simulink model "atrias_original"  (R2017a)
settings: Solver=ode45  StartTime=0.0  StopTime=sim_t  RelTol=1e-6  EnableMultiTasking=on
values from neighbouring files (symbols this model uses):
  N = grid_slice*1000    [createGrid.m]
  nm = fn_set_vnmc_params(sm, sample_time)    [kernel_scores_NM_mismatch.m]    (also in main_ATRIAS_cluster.m)
  nmc_BLCtrlPar = nmc.BLCtrlPar    [kernel_scores_NM_mismatch.m]    (also in main_ATRIAS_cluster.m)
  nmc_FPCtrlPar = nmc.FPCtrlPar    [kernel_scores_NM_mismatch.m]    (also in main_ATRIAS_cluster.m)
  nmc_LLCtrlPar = nmc.LLCtrlPar    [kernel_scores_NM_mismatch.m]    (also in main_ATRIAS_cluster.m)
  nmc_StCtrlPar = nmc.StCtrlPar    [kernel_scores_NM_mismatch.m]    (also in main_ATRIAS_cluster.m)
  nmc_SwCtrlPar = nmc.SwCtrlPar    [kernel_scores_NM_mismatch.m]    (also in main_ATRIAS_cluster.m)
  nmc_TrCtrlPar = nmc.TrCtrlPar    [kernel_scores_NM_mismatch.m]    (also in main_ATRIAS_cluster.m)
  nStep_switchCtrl = 10    [main_ATRIAS_cluster.m]
  nStep_thr = 1000    [createSimInitial.m]    (also in main_ATRIAS_cluster.m)
  rc_CtrlPar = [rc.k_placement, rc.T_step, rc.Cd, rc.kpt, rc.kdt, rc.desired_theta, rc.desired_z, rc.kpz, rc.kdz]    [kernel_scores_NM_mismatch.m]    (also in main_ATRIAS_cluster.m)
  sm = fn_set_MechParams(sm)    [kernel_scores_NM_mismatch.m]    (also in main_ATRIAS_cluster.m = fn_set_MechParams(sm,perturb))
  test_VNMC = 1    [createSimInitial.m]    (also in main_ATRIAS_cluster.m = 0)
undefined symbols (not defined in the file or in its folder): delta_phi_max, delta_phi_max_buffer, delta_phi_min, DiscIntNeverNeededParam, Discrete, idc, initial_dx_estimate, initial_dy_estimate, initial_dz_estimate, initial_z_estimate, kd_shin_max, kd_shin_min, kd_splay_max, kd_splay_min, kd_thigh_max, kd_thigh_min, kp_shin_max, kp_shin_min, kp_splay_max, kp_splay_min, kp_thigh_max, kp_thigh_min, mc, min_splay_angle, min_splay_buffer, phi_shin_max, phi_shin_max_buffer, phi_shin_min, phi_shin_min_buffer, phi_thigh_max, phi_thigh_max_buffer, phi_thigh_min, phi_thigh_min_buffer, rad, rc, s, sample_time, sgn, sim_d, t_friction, Time, X, Y, Z
libraries: sm_lib x202, nesl_utility x122, simulink x77, simulink_extras x24, fl_lib x16, mblibv1 x4, ctrlSharedLib x4, commnoisgen2 x1, dspswit3 x1
(part 8 of 17)

== system atrias_original/ATRIAS_sim/Mechanical System Layer/R Hip Shaft/Frame Data ==
  Kinematic Data : ToWorkspace  VariableName=r_hip_out  SampleTime=sm.output_sample_time
      settings: Save2DSignal=2-D array (concatenate along first dimension)
  Mux : Mux
  PS-Simulink Converter{,1..3} (4 alike) : nesl_utility/PS-Simulink Converter  PhysicalDomain=network_engine_domain  SubClassName=ps_output  LeftPortType=input  RightPortType=output  PseudoPeriodic=off  Frequencies=[]  Unit=1  AffineConversion=off
  Transform Sensor : sm_lib/Frames and Transforms/Transform Sensor  MeasurementFrame=World  SenseAngle=off  SenseAxis=off  SenseAngle1=off  SenseAngle2=off  SenseAngle3=off  SenseQ=on  SenseR=off  SenseOmegaX=off  SenseOmegaY=off  SenseOmegaZ=off  SenseOmega1=off  SenseOmega2=off  SenseOmega3=off  SenseQDot=off  SenseRDot=off  SenseAlphaX=off  SenseAlphaY=off  SenseAlphaZ=off  SenseAlpha1=off  SenseAlpha2=off  SenseAlpha3=off  SenseQDDot=off  SenseRDDot=off  SenseX=on  SenseY=on  SenseZ=on  SenseRad=off  SenseAzim=off  SenseDist=off  SenseInc=off  SenseXDot=off  SenseYDot=off  SenseZDot=off  SenseRadDot=off  SenseAzimDot=off  SenseDistDot=off  SenseIncDot=off  SenseXDDot=off  SenseYDDot=off  SenseZDDot=off  SenseRadDDot=off  SenseAzimDDot=off  SenseDistDDot=off  SenseIncDDot=off
  World Frame : sm_lib/Frames and Transforms/World Frame
  Frame : PMIOPort  Port=1  Side=Left
  wires:
  Mux/1 -> Kinematic Data/1
  PS-Simulink Converter/1 -> Mux/1
  PS-Simulink Converter1/1 -> Mux/2
  PS-Simulink Converter2/1 -> Mux/3
  PS-Simulink Converter3/1 -> Mux/4
  connections:
  PS-Simulink Converter3/LConn1 -- Transform Sensor/RConn5
  PS-Simulink Converter2/LConn1 -- Transform Sensor/RConn4
  PS-Simulink Converter1/LConn1 -- Transform Sensor/RConn3
  PS-Simulink Converter/LConn1 -- Transform Sensor/RConn2
  Transform Sensor/RConn1 -- Frame/RConn1
  Transform Sensor/LConn1 -- World Frame/RConn1

== system atrias_original/ATRIAS_sim/Mechanical System Layer/R Leg/Angle Range Map ==
  "[-pi, pi]" : Inport
  Constant : Constant  Value=2*pi
  Sum3 : Sum  Inputs=|++
  Switch : Switch  ZeroCross=off
  "[0,2*pi]" : Outport
  wires:
  "[-pi, pi]"/1 -> Sum3/1, Switch/1, Switch/2
  Sum3/1 -> Switch/3
  Constant/1 -> Sum3/2
  Switch/1 -> "[0,2*pi]"/1

== system atrias_original/ATRIAS_sim/Mechanical System Layer/R Leg/Angle Range Map1 ==
  "[-pi, pi]" : Inport
  Constant : Constant  Value=2*pi
  Sum3 : Sum  Inputs=|++
  Switch : Switch  ZeroCross=off
  "[0,2*pi]" : Outport
  wires:
  Switch/1 -> "[0,2*pi]"/1
  Constant/1 -> Sum3/2
  Sum3/1 -> Switch/3
  "[-pi, pi]"/1 -> Switch/2, Switch/1, Sum3/1

== system atrias_original/ATRIAS_sim/Mechanical System Layer/R Leg/Four Bar Link ==
  CS1 to CS2 : sm_lib/Frames and Transforms/Rigid Transform  TranslationMethod=Cartesian  TranslationStandardOffset=0  TranslationLengthUnit=m  TranslationStandardAxis=+Z  TranslationCartesianOffset=[0 -sm.l_seg 0]  TranslationROffset=0  TranslationROffsetUnits=m  TranslationZOffset=0  TranslationZOffsetUnits=m  TranslationThetaOffset=0  TranslationThetaOffsetUnits=deg  RotationMethod=None  RotationAngleUnits=deg  RotationStandardAxis=+Z  RotationAngle=0  RotationArbitraryAxis=[0 0 1]  FollAlignAxisA=+X  BaseAlignAxisA=+Y  FollAlignAxisB=+Y  BaseAlignAxisB=+Z  RotationSequenceAxes=FollowerAxes  RotationSequence=XYX  RotationSequenceAngles=[0 0 0]  RotationSequenceAnglesUnits=deg  RotationMatrix=[1 0 0; 0 1 0; 0 0 1]
  Frame Data : Subsystem
  Solid : sm_lib/Body Elements/Solid  InertiaType=Custom  Mass=sm.m_fblink  MassUnits=kg  CenterOfMass=sm.com_fblink  CenterOfMassUnits=m  MomentsOfInertia=sm.i_fblink_moments  MomentsOfInertiaUnits=kg*m^2  ProductsOfInertia=sm.i_fblink_products  ProductsOfInertiaUnits=kg*m^2  DensityBased=on  Density=1000  DensityUnits=kg/(m^3)  DoExposeReferenceFrame=on  SerializedFrames=<Frames/>  GraphicType=FromGeometry  MarkerShape=Sphere  MarkerSize=10  MarkerSizeUnits=m  GraphicVisPropType=AdvancedVisualProperties  GraphicDiffuseColor=sm.fblink_color_d  GraphicSpecularColor=[0.5 0.5 0.5 1.0]  GraphicAmbientColor=[sm.fblink_color_d*0.5 1.0]  GraphicEmissiveColor=[0.0 0.0 0.0 1.0]  GraphicShininess=128  GraphicOpacity=1.0  GeometryShape=FromFile  RectangleSize=[1 1]  RectangleSizeUnits=m  BrickDimensions="[0.1  1 0.1]"  BrickDimensionUnits=m  CylinderRadius=1  CylinderRadiusUnits=m  CylinderLength=1  CylinderLengthUnits=m  SphereRadius=1  SphereRadiusUnits=m  EllipsoidRadii=[1 1 1]  EllipsoidRadiiUnits=m  ExtrusionCrossSection=[1 1; -1 1; -1 -1; 1 -1]  ExtrusionCrossSectionUnits=m  ExtrusionLength=1  ExtrusionLengthUnits=m  PolygonNumSides=3  PolygonOuterRadius=1  PolygonOuterRadiusUnits=m  ExtGeomFileType=STL  ExtGeomFileName=../models/four_bar_link.stl  ExtGeomFileUnits=m  RevolutionCrossSection=[1 1; 1 -1; 2 -1; 2 1]  RevolutionCrossSectionUnits=m  RevolutionExtent=Full  RevolutionAngle=180  RevolutionAngleUnits=deg
  CS1 : PMIOPort  Port=1  Side=Left
  CS2 : PMIOPort  Port=2  Side=Right
  connections:
  CS2/RConn1 -- CS1 to CS2/RConn1
  Solid/RConn1 -- CS1/RConn1 -- Frame Data/LConn1 -- CS1 to CS2/LConn1

== system atrias_original/ATRIAS_sim/Mechanical System Layer/R Leg/Lower Leg ==
  CS1 to CS2 : sm_lib/Frames and Transforms/Rigid Transform  TranslationMethod=Cartesian  TranslationStandardOffset=0  TranslationLengthUnit=m  TranslationStandardAxis=+Z  TranslationCartesianOffset=[0 -sm.lowerleg_12 0]  TranslationROffset=0  TranslationROffsetUnits=m  TranslationZOffset=0  TranslationZOffsetUnits=m  TranslationThetaOffset=0  TranslationThetaOffsetUnits=deg  RotationMethod=None  RotationAngleUnits=deg  RotationStandardAxis=+Z  RotationAngle=0  RotationArbitraryAxis=[0 0 1]  FollAlignAxisA=+X  BaseAlignAxisA=+Y  FollAlignAxisB=+Y  BaseAlignAxisB=+Z  RotationSequenceAxes=FollowerAxes  RotationSequence=XYX  RotationSequenceAngles=[0 0 0]  RotationSequenceAnglesUnits=deg  RotationMatrix=[1 0 0; 0 1 0; 0 0 1]
  CS1 to CS3 : sm_lib/Frames and Transforms/Rigid Transform  TranslationMethod=Cartesian  TranslationStandardOffset=0  TranslationLengthUnit=m  TranslationStandardAxis=+Z  TranslationCartesianOffset=[0 -sm.l_seg 0]  TranslationROffset=0  TranslationROffsetUnits=m  TranslationZOffset=0  TranslationZOffsetUnits=m  TranslationThetaOffset=0  TranslationThetaOffsetUnits=deg  RotationMethod=None  RotationAngleUnits=deg  RotationStandardAxis=+Z  RotationAngle=0  RotationArbitraryAxis=[0 0 1]  FollAlignAxisA=+X  BaseAlignAxisA=+Y  FollAlignAxisB=+Y  BaseAlignAxisB=+Z  RotationSequenceAxes=FollowerAxes  RotationSequence=XYX  RotationSequenceAngles=[0 0 0]  RotationSequenceAnglesUnits=deg  RotationMatrix=[1 0 0; 0 1 0; 0 0 1]
  Frame Data : Subsystem
  Solid : sm_lib/Body Elements/Solid  InertiaType=Custom  Mass=sm.m_lowerleg  MassUnits=kg  CenterOfMass=sm.com_lowerleg  CenterOfMassUnits=m  MomentsOfInertia=sm.i_lowerleg_moments  MomentsOfInertiaUnits=kg*m^2  ProductsOfInertia=sm.i_lowerleg_products  ProductsOfInertiaUnits=kg*m^2  DensityBased=on  Density=1000  DensityUnits=kg/(m^3)  DoExposeReferenceFrame=on  SerializedFrames=<Frames/>  GraphicType=FromGeometry  MarkerShape=Sphere  MarkerSize=10  MarkerSizeUnits=m  GraphicVisPropType=AdvancedVisualProperties  GraphicDiffuseColor=sm.lowerleg_color_d  GraphicSpecularColor=[0.5 0.5 0.5 1.0]  GraphicAmbientColor=[sm.lowerleg_color_d*0.5 1.0]  GraphicEmissiveColor=[0.0 0.0 0.0 1.0]  GraphicShininess=128  GraphicOpacity=1.0  GeometryShape=FromFile  RectangleSize=[1 1]  RectangleSizeUnits=m  BrickDimensions=[0.1 1 0.1]  BrickDimensionUnits=m  CylinderRadius=1  CylinderRadiusUnits=m  CylinderLength=1  CylinderLengthUnits=m  SphereRadius=1  SphereRadiusUnits=m  EllipsoidRadii=[1 1 1]  EllipsoidRadiiUnits=m  ExtrusionCrossSection=[1 1; -1 1; -1 -1; 1 -1]  ExtrusionCrossSectionUnits=m  ExtrusionLength=1  ExtrusionLengthUnits=m  PolygonNumSides=3  PolygonOuterRadius=1  PolygonOuterRadiusUnits=m  ExtGeomFileType=STL  ExtGeomFileName=../models/lower_leg.stl  ExtGeomFileUnits=m  RevolutionCrossSection=[1 1; 1 -1; 2 -1; 2 1]  RevolutionCrossSectionUnits=m  RevolutionExtent=Full  RevolutionAngle=180  RevolutionAngleUnits=deg
  CS1 : PMIOPort  Port=1  Side=Left
  CS2 : PMIOPort  Port=2  Side=Right
  CS3 : PMIOPort  Port=3  Side=Right
  connections:
  CS3/RConn1 -- CS1 to CS3/RConn1
  CS1 to CS3/LConn1 -- CS1 to CS2/LConn1 -- Solid/RConn1 -- Frame Data/LConn1 -- CS1/RConn1
  CS2/RConn1 -- CS1 to CS2/RConn1

== system atrias_original/ATRIAS_sim/Mechanical System Layer/R Leg/Mechanical Limits ==
  note: Thigh-Shin Flexion Collision
  note: Thigh-Shin Collision
  note: Mechanical Limits Model
  dphi_shin : Inport
  phi_shin : Inport  Port=2
  dphi_thigh : Inport  Port=3
  phi_thigh : Inport  Port=4
  Compare To Constant5 : simulink/Logic and Bit Operations/Compare To Constant  relop=<=  const=sm.phi_max_collision  OutDataTypeStr=boolean  ZeroCross=off
  Compare To Zero{,1..5} (6 alike) : simulink/Logic and Bit Operations/Compare To Zero  relop=<=  OutDataTypeStr=boolean  ZeroCross=off
  Constant : Constant  Value=sm.delta_phi_min
  Constant1 : Constant  Value=sm.phi_shin_max
  Constant2 : Constant  Value=sm.phi_thigh_min
  Constant3 : Constant  Value=sm.delta_phi_max
  Constant4 : Constant  Value=sm.phi_shin_min
  Constant5 : Constant  Value=sm.phi_thigh_max
  Enabled Subsystem : Subsystem  TreatAsAtomicUnit=on
  Gain : Gain  Gain=-1
  Gain1 : Gain  Gain=-1
  Gain2 : Gain  Gain=-1
  Logical Operator : Logic  Operator=OR  Inputs=1  AllPortsSameDT=off  OutDataTypeStr=boolean
  Mux : Mux  Inputs=6
  Shin Max Collision Model : Subsystem
  Shin Min Collision Model : Subsystem
  Stop Simulation6 : Stop
  Sum{1..3,5,7} (5 alike) : Sum  Inputs=-+|
  Sum10 : Sum  Inputs=+-|
  Sum11 : Sum  Inputs=-|+
  Sum4 : Sum  Inputs=+-|
  Sum6 : Sum  Inputs=+|-
  Sum8 : Sum  Inputs=+-|
  Sum9 : Sum  Inputs=-|+
  Thigh Max Collision Model : Subsystem
  Thigh Min Collision Model : Subsystem
  Thigh-Shin Collision Model : Subsystem
  Thigh-Shin Collision Model1 : Subsystem
  tau_shin_col : Outport
  tau_thigh_shin_col : Outport  Port=2
  tau_thigh_col : Outport  Port=3
  wires:
  Compare To Constant5/1 -> Logical Operator/1, Enabled Subsystem/1(Col_Flags)
  Sum4/1 -> Shin Max Collision Model/1(phi [rad]), Compare To Zero1/1, [col_r_shin_max]
  Sum10/1 -> [col_r_thigh_max], Compare To Zero5/1, Thigh Max Collision Model/1(phi [rad])
  Logical Operator/1 -> Enabled Subsystem/Enable, Stop Simulation6/1
  Mux/1 -> Compare To Constant5/1
  [col_r_leg_flexion] -> Mux/6
  [col_r_leg_extension] -> Mux/5
  [col_r_shin_min] -> Mux/4
  [col_r_shin_max] -> Mux/3
  [col_r_thigh_min] -> Mux/2
  [col_r_thigh_max] -> Mux/1
  Thigh Max Collision Model/1(tau_interaction[Nm]) -> Sum11/1
  Gain1/1 -> Thigh Max Collision Model/2(vphi [rad/s])
  Thigh Min Collision Model/1(tau_interaction[Nm]) -> Sum11/2
  Sum11/1 -> tau_thigh_col/1
  Compare To Zero5/1 -> Thigh Max Collision Model/Enable
  Constant5/1 -> Sum10/1
  Sum6/1 -> tau_thigh_shin_col/1
  Shin Min Collision Model/1(tau_interaction[Nm]) -> Sum9/2
  Shin Max Collision Model/1(tau_interaction[Nm]) -> Sum9/1
  Sum9/1 -> tau_shin_col/1
  dphi_shin/1 -> Shin Min Collision Model/2(vphi [rad/s]), Gain/1, Sum2/2
  Sum7/1 -> Shin Min Collision Model/1(phi [rad]), Compare To Zero4/1, [col_r_shin_min]
  Constant4/1 -> Sum7/1
  Compare To Zero4/1 -> Shin Min Collision Model/Enable
  Gain2/1 -> Thigh-Shin Collision Model1/2(vphi [rad/s])
  Thigh-Shin Collision Model1/1(tau_interaction[Nm]) -> Sum6/2
  Thigh-Shin Collision Model/1(tau_interaction[Nm]) -> Sum6/1
  Sum8/1 -> Thigh-Shin Collision Model1/1(delta_phi [rad]), Compare To Zero3/1, [col_r_leg_flexion]
  Constant3/1 -> Sum8/1
  Compare To Zero3/1 -> Thigh-Shin Collision Model1/Enable
  Compare To Zero2/1 -> Thigh Min Collision Model/Enable
  Gain/1 -> Shin Max Collision Model/2(vphi [rad/s])
  Sum5/1 -> Thigh Min Collision Model/1(phi [rad]), Compare To Zero2/1, [col_r_thigh_min]
  Constant2/1 -> Sum5/1
  dphi_thigh/1 -> Sum2/1, Gain1/1, Thigh Min Collision Model/2(vphi [rad/s])
  phi_thigh/1 -> Sum1/1, Sum5/2, Sum10/2
  Constant1/1 -> Sum4/1
  Compare To Zero1/1 -> Shin Max Collision Model/Enable
  Sum3/1 -> Thigh-Shin Collision Model/1(delta_phi [rad]), Compare To Zero/1, [col_r_leg_extension]
  Constant/1 -> Sum3/1
  Sum2/1 -> Thigh-Shin Collision Model/2(vphi [rad/s]), Gain2/1
  phi_shin/1 -> Sum4/2, Sum7/2, Sum1/2
  Sum1/1 -> Sum3/2, Sum8/2
  Compare To Zero/1 -> Thigh-Shin Collision Model/Enable

== system atrias_original/ATRIAS_sim/Mechanical System Layer/R Leg/Shin ==
  CS1 to CS2 : sm_lib/Frames and Transforms/Rigid Transform  TranslationMethod=Cartesian  TranslationStandardOffset=0  TranslationLengthUnit=m  TranslationStandardAxis=+Z  TranslationCartesianOffset=[0 -sm.shin_12 0]  TranslationROffset=0  TranslationROffsetUnits=m  TranslationZOffset=0  TranslationZOffsetUnits=m  TranslationThetaOffset=0  TranslationThetaOffsetUnits=deg  RotationMethod=None  RotationAngleUnits=deg  RotationStandardAxis=+Z  RotationAngle=0  RotationArbitraryAxis=[0 0 1]  FollAlignAxisA=+X  BaseAlignAxisA=+Y  FollAlignAxisB=+Y  BaseAlignAxisB=+Z  RotationSequenceAxes=FollowerAxes  RotationSequence=XYX  RotationSequenceAngles=[0 0 0]  RotationSequenceAnglesUnits=deg  RotationMatrix=[1 0 0; 0 1 0; 0 0 1]
  Frame Data : Subsystem
  Solid : sm_lib/Body Elements/Solid  InertiaType=Custom  Mass=sm.m_shin  MassUnits=kg  CenterOfMass=sm.com_shin  CenterOfMassUnits=m  MomentsOfInertia=sm.i_shin_moments  MomentsOfInertiaUnits=kg*m^2  ProductsOfInertia=sm.i_shin_products  ProductsOfInertiaUnits=kg*m^2  DensityBased=on  Density=1000  DensityUnits=kg/(m^3)  DoExposeReferenceFrame=on  SerializedFrames=<Frames/>  GraphicType=FromGeometry  MarkerShape=Sphere  MarkerSize=10  MarkerSizeUnits=m  GraphicVisPropType=AdvancedVisualProperties  GraphicDiffuseColor=sm.shin_color_d  GraphicSpecularColor=[0.5 0.5 0.5 1.0]  GraphicAmbientColor=[sm.shin_color_d*0.5 1.0]  GraphicEmissiveColor=[0.0 0.0 0.0 1.0]  GraphicShininess=128  GraphicOpacity=1.0  GeometryShape=FromFile  RectangleSize=[1 1]  RectangleSizeUnits=m  BrickDimensions=[1 1 1]  BrickDimensionUnits=m  CylinderRadius=1  CylinderRadiusUnits=m  CylinderLength=1  CylinderLengthUnits=m  SphereRadius=1  SphereRadiusUnits=m  EllipsoidRadii=[1 1 1]  EllipsoidRadiiUnits=m  ExtrusionCrossSection=[1 1; -1 1; -1 -1; 1 -1]  ExtrusionCrossSectionUnits=m  ExtrusionLength=1  ExtrusionLengthUnits=m  PolygonNumSides=3  PolygonOuterRadius=1  PolygonOuterRadiusUnits=m  ExtGeomFileType=STL  ExtGeomFileName=../models/shin.stl  ExtGeomFileUnits=m  RevolutionCrossSection=[1 1; 1 -1; 2 -1; 2 1]  RevolutionCrossSectionUnits=m  RevolutionExtent=Full  RevolutionAngle=180  RevolutionAngleUnits=deg
  CS1 : PMIOPort  Port=1  Side=Left
  CS2 : PMIOPort  Port=2  Side=Right
  connections:
  CS1 to CS2/LConn1 -- CS1/RConn1 -- Frame Data/LConn1 -- Solid/RConn1
  CS2/RConn1 -- CS1 to CS2/RConn1

== system atrias_original/ATRIAS_sim/Mechanical System Layer/R Leg/Shin SEA ==
  note: Shin SEA Mechanics
  Shin Gear Torque [Nm] : Inport
  Shin Joint [rad rad/s] : Inport  Port=2
  Continuous Angle : mblibv1/Utilities/Continuous Angle  rad=rad  rads=rad/s
      settings: SourceProductName=Simscape Multibody  SourceProductBaseCode=MS
  Demux : Demux  Outputs=2
  Gain : Gain  Gain=sm.k_leg_spring
  Gain1 : Gain  Gain=sm.b_leg_spring
  Initial Gear Angle : Constant  Value=sm.shin_initial_r
  Inverse Gear Ratio1 : Gain  Gain=1/sm.N
  Inverse Gear Ratio2 : Gain  Gain=sm.Kt_leg
  Inverse Gear Ratio3 : Gain  Gain=1/sm.Kt_leg
  Motor Direction : Gain  Gain=-1
  Motor Efficiency : Gain  Gain=sm.mu_motor
  Motor Controller : Subsystem  Commented=on
  Motor Electromagnetism : Subsystem  Commented=on
  Rotor Damping : Gain  Gain=sm.b_rotor
  Rotor and Gearing : Subsystem
  Sum : Sum  Inputs=++|
  Sum2 : Sum  Inputs=+|-
  Sum3 : Sum  Inputs=|+-
  Sum4 : Sum  Inputs=+|-
  Sum5 : Sum  Inputs=|++
  Torque Limiter (outside) 2 : Saturate  UpperLimit=sm.LEG_MTR_MAX_TORQUE  LowerLimit=-sm.LEG_MTR_MAX_TORQUE  ZeroCross=off
      settings: AttributesFormatString=Hi: %<UpperLimit>\nLo: %<LowerLimit>
  Rotor Joint Conn : PMIOPort  Port=1  Side=Left
  Shin Joint Torque [Nm] : Outport
  Shin Gear [rad] : Outport  Port=2
  wires:
  Sum2/1 -> Gain/1
  Gain/1 -> Sum5/1  "tau_load"
  Gain1/1 -> Sum5/2
  Sum4/1 -> Gain1/1
  Shin Joint [rad rad/s]/1 -> Demux/1
  Demux/1 -> Sum2/2
  Demux/2 -> Sum4/2
  Initial Gear Angle/1 -> Sum/1
  Sum/1 -> Sum2/1, Shin Gear [rad]/1
  Shin Gear Torque [Nm]/1 -> Motor Direction/1
  Sum3/1 -> Motor Efficiency/1
  Rotor Damping/1 -> Sum3/2
  Inverse Gear Ratio3/1 -> Inverse Gear Ratio2/1
  Inverse Gear Ratio2/1 -> Sum3/1
  Motor Controller/1(Voltage [V]) -> Motor Electromagnetism/1(Voltage [V])
  Motor Electromagnetism/1(Current [A]) -> Motor Controller/2(Measured Current [A])
  Inverse Gear Ratio1/1 -> Inverse Gear Ratio3/1
  Motor Efficiency/1 -> Rotor and Gearing/1(Rotor Torque [Nm])
  Rotor and Gearing/3(Rotor Velocity [rad/s]) -> Rotor Damping/1
  Torque Limiter (outside) 2/1 -> Inverse Gear Ratio1/1
  Sum5/1 -> Rotor and Gearing/2(Spring Torque [Nm]), Shin Joint Torque [Nm]/1
  Rotor and Gearing/1(Gearhead Position [rad]) -> Continuous Angle/1
  Rotor and Gearing/2(Gearhead Velocity [rad/s]) -> Sum4/1, Continuous Angle/2
  Continuous Angle/1 -> Sum/2
  Motor Direction/1 -> Torque Limiter (outside) 2/1
  connections:
  Rotor and Gearing/LConn1 -- Rotor Joint Conn/RConn1

== system atrias_original/ATRIAS_sim/Mechanical System Layer/R Leg/Thigh ==
  CS1 to CS2 : sm_lib/Frames and Transforms/Rigid Transform  TranslationMethod=Cartesian  TranslationStandardOffset=0  TranslationLengthUnit=m  TranslationStandardAxis=+Z  TranslationCartesianOffset=[0 -sm.l_seg 0]  TranslationROffset=0  TranslationROffsetUnits=m  TranslationZOffset=0  TranslationZOffsetUnits=m  TranslationThetaOffset=0  TranslationThetaOffsetUnits=deg  RotationMethod=None  RotationAngleUnits=deg  RotationStandardAxis=+Z  RotationAngle=0  RotationArbitraryAxis=[0 0 1]  FollAlignAxisA=+X  BaseAlignAxisA=+Y  FollAlignAxisB=+Y  BaseAlignAxisB=+Z  RotationSequenceAxes=FollowerAxes  RotationSequence=XYX  RotationSequenceAngles=[0 0 0]  RotationSequenceAnglesUnits=deg  RotationMatrix=[1 0 0; 0 1 0; 0 0 1]
  Frame Data : Subsystem
  Solid : sm_lib/Body Elements/Solid  InertiaType=Custom  Mass=sm.m_thigh  MassUnits=kg  CenterOfMass=sm.com_thigh  CenterOfMassUnits=m  MomentsOfInertia=sm.i_thigh_moments  MomentsOfInertiaUnits=kg*m^2  ProductsOfInertia=sm.i_thigh_products  ProductsOfInertiaUnits=kg*m^2  DensityBased=on  Density=1000  DensityUnits=kg/(m^3)  DoExposeReferenceFrame=on  SerializedFrames=<Frames/>  GraphicType=FromGeometry  MarkerShape=Sphere  MarkerSize=10  MarkerSizeUnits=m  GraphicVisPropType=AdvancedVisualProperties  GraphicDiffuseColor=sm.thigh_color_d  GraphicSpecularColor=[0.5 0.5 0.5 1.0]  GraphicAmbientColor=[sm.thigh_color_d*0.5 1.0]  GraphicEmissiveColor=[0.0 0.0 0.0 1.0]  GraphicShininess=128  GraphicOpacity=1.0  GeometryShape=FromFile  RectangleSize=[1 1]  RectangleSizeUnits=m  BrickDimensions=[1 1 1]  BrickDimensionUnits=m  CylinderRadius=1  CylinderRadiusUnits=m  CylinderLength=1  CylinderLengthUnits=m  SphereRadius=1  SphereRadiusUnits=m  EllipsoidRadii=[1 1 1]  EllipsoidRadiiUnits=m  ExtrusionCrossSection=[1 1; -1 1; -1 -1; 1 -1]  ExtrusionCrossSectionUnits=m  ExtrusionLength=1  ExtrusionLengthUnits=m  PolygonNumSides=3  PolygonOuterRadius=1  PolygonOuterRadiusUnits=m  ExtGeomFileType=STL  ExtGeomFileName=../models/thigh.stl  ExtGeomFileUnits=m  RevolutionCrossSection=[1 1; 1 -1; 2 -1; 2 1]  RevolutionCrossSectionUnits=m  RevolutionExtent=Full  RevolutionAngle=180  RevolutionAngleUnits=deg
  CS1 : PMIOPort  Port=1  Side=Left
  CS2 : PMIOPort  Port=2  Side=Right
  connections:
  CS2/RConn1 -- CS1 to CS2/RConn1
  CS1 to CS2/LConn1 -- Solid/RConn1 -- Frame Data/LConn1 -- CS1/RConn1

== system atrias_original/ATRIAS_sim/Mechanical System Layer/R Leg/Thigh SEA ==
  note: Thigh SEA Mechanics
  Thigh Gear Torque [Nm] : Inport
  Thigh Joint [rad rad/s] : Inport  Port=2
  Continuous Angle : mblibv1/Utilities/Continuous Angle  rad=rad  rads=rad/s
      settings: SourceProductName=Simscape Multibody  SourceProductBaseCode=MS
  Demux : Demux  Outputs=2
  Gain : Gain  Gain=sm.k_leg_spring
  Gain1 : Gain  Gain=sm.b_leg_spring
  Initial Gear Angle : Constant  Value=sm.thigh_initial_r
  Inverse Gear Ratio1 : Gain  Gain=1/sm.N
  Inverse Gear Ratio2 : Gain  Gain=sm.Kt_leg
  Inverse Gear Ratio3 : Gain  Gain=1/sm.Kt_leg
  Motor Direction : Gain  Gain=-1
  Motor Efficiency : Gain  Gain=sm.mu_motor
  Motor Controller : Subsystem  Commented=on
  Motor Electromagnetism : Subsystem  Commented=on
  Rotor Damping : Gain  Gain=sm.b_rotor
  Rotor and Gearing : Subsystem
  Sum : Sum  Inputs=++|
  Sum2 : Sum  Inputs=+|-
  Sum3 : Sum  Inputs=|+-
  Sum4 : Sum  Inputs=+|-
  Sum5 : Sum  Inputs=|++
  Torque Limiter (outside) 2 : Saturate  UpperLimit=sm.LEG_MTR_MAX_TORQUE  LowerLimit=-sm.LEG_MTR_MAX_TORQUE  ZeroCross=off
      settings: AttributesFormatString=Hi: %<UpperLimit>\nLo: %<LowerLimit>
  Rotor Joint Conn : PMIOPort  Port=1  Side=Left
  Thigh Joint Torque [Nm] : Outport
  Thigh Gear [rad] : Outport  Port=2
  wires:
  Sum2/1 -> Gain/1
  Sum3/1 -> Motor Efficiency/1
  Rotor Damping/1 -> Sum3/2
  Gain/1 -> Sum5/1  "tau_load"
  Gain1/1 -> Sum5/2
  Sum4/1 -> Gain1/1
  Thigh Joint [rad rad/s]/1 -> Demux/1
  Demux/1 -> Sum2/2
  Demux/2 -> Sum4/2
  Inverse Gear Ratio3/1 -> Inverse Gear Ratio2/1
  Inverse Gear Ratio2/1 -> Sum3/1
  Initial Gear Angle/1 -> Sum/1
  Sum/1 -> Thigh Gear [rad]/1, Sum2/1
  Continuous Angle/1 -> Sum/2
  Rotor and Gearing/1(Gearhead Position [rad]) -> Continuous Angle/1
  Motor Controller/1(Voltage [V]) -> Motor Electromagnetism/1(Voltage [V])
  Motor Electromagnetism/1(Current [A]) -> Motor Controller/2(Measured Current [A])
  Thigh Gear Torque [Nm]/1 -> Motor Direction/1
  Inverse Gear Ratio1/1 -> Inverse Gear Ratio3/1
  Motor Efficiency/1 -> Rotor and Gearing/1(Rotor Torque [Nm])
  Rotor and Gearing/2(Gearhead Velocity [rad/s]) -> Sum4/1, Continuous Angle/2
  Sum5/1 -> Thigh Joint Torque [Nm]/1, Rotor and Gearing/2(Spring Torque [Nm])
  Rotor and Gearing/3(Rotor Velocity [rad/s]) -> Rotor Damping/1
  Torque Limiter (outside) 2/1 -> Inverse Gear Ratio1/1
  Motor Direction/1 -> Torque Limiter (outside) 2/1
  connections:
  Rotor and Gearing/LConn1 -- Rotor Joint Conn/RConn1

== system atrias_original/ATRIAS_sim/Mechanical System Layer/Right Hip Roll Joint/Mechanical Limits  ==
  vphi : Inport
  phi : Inport  Port=2
  Compare To Constant5 : simulink/Logic and Bit Operations/Compare To Constant  relop=<=  const=sm.phi_max_collision  OutDataTypeStr=boolean  ZeroCross=off
  Compare To Zero1 : simulink/Logic and Bit Operations/Compare To Zero  relop=<=  OutDataTypeStr=boolean  ZeroCross=off
  Compare To Zero2 : simulink/Logic and Bit Operations/Compare To Zero  relop=<=  OutDataTypeStr=boolean  ZeroCross=off
  Constant1 : Constant  Value=sm.phi_roll_min
  Constant2 : Constant  Value=sm.phi_roll_max
  Enabled Subsystem : Subsystem  TreatAsAtomicUnit=on
  Gain2 : Gain  Gain=-1
  Logical Operator : Logic  Operator=OR  Inputs=1  AllPortsSameDT=off  OutDataTypeStr=boolean
  Mux : Mux  Inputs=2
  Roll Max Collision Model : Subsystem
  Roll Min Collision Model : Subsystem
  Stop Simulation6 : Stop
  Sum1 : Sum  Inputs=-+|
  Sum11 : Sum  Inputs=-|+
  Sum5 : Sum  Inputs=+-|
  tau_reaction : Outport
  wires:
  Sum1/1 -> [col_hip_min], Compare To Zero1/1, Roll Min Collision Model/1(phi [rad])
  Roll Min Collision Model/1(tau_interaction[Nm]) -> Sum11/2
  Compare To Zero1/1 -> Roll Min Collision Model/Enable
  phi/1 -> Sum1/2, Sum5/2
  Logical Operator/1 -> Stop Simulation6/1, Enabled Subsystem/Enable
  [col_hip_max] -> Mux/1
  Mux/1 -> Compare To Constant5/1
  [col_hip_min] -> Mux/2
  Sum11/1 -> tau_reaction/1
  Constant1/1 -> Sum1/1
  Compare To Constant5/1 -> Enabled Subsystem/1(Col_Flags), Logical Operator/1
  Constant2/1 -> Sum5/1
  Sum5/1 -> [col_hip_max], Compare To Zero2/1, Roll Max Collision Model/1(phi [rad])
  Compare To Zero2/1 -> Roll Max Collision Model/Enable
  Roll Max Collision Model/1(tau_interaction[Nm]) -> Sum11/1
  vphi/1 -> Roll Min Collision Model/2(vphi [rad/s]), Gain2/1
  Gain2/1 -> Roll Max Collision Model/2(vphi [rad/s])

== system atrias_original/ATRIAS_sim/Mechanical System Layer/Torso/Frame Data ==
  Kinematic Data : ToWorkspace  VariableName=torso_out  SampleTime=sm.output_sample_time
      settings: Save2DSignal=2-D array (concatenate along first dimension)
  Mux : Mux
  PS-Simulink Converter{,1..3} (4 alike) : nesl_utility/PS-Simulink Converter  PhysicalDomain=network_engine_domain  SubClassName=ps_output  LeftPortType=input  RightPortType=output  PseudoPeriodic=off  Frequencies=[]  Unit=1  AffineConversion=off
  Transform Sensor : sm_lib/Frames and Transforms/Transform Sensor  MeasurementFrame=World  SenseAngle=off  SenseAxis=off  SenseAngle1=off  SenseAngle2=off  SenseAngle3=off  SenseQ=on  SenseR=off  SenseOmegaX=off  SenseOmegaY=off  SenseOmegaZ=off  SenseOmega1=off  SenseOmega2=off  SenseOmega3=off  SenseQDot=off  SenseRDot=off  SenseAlphaX=off  SenseAlphaY=off  SenseAlphaZ=off  SenseAlpha1=off  SenseAlpha2=off  SenseAlpha3=off  SenseQDDot=off  SenseRDDot=off  SenseX=on  SenseY=on  SenseZ=on  SenseRad=off  SenseAzim=off  SenseDist=off  SenseInc=off  SenseXDot=off  SenseYDot=off  SenseZDot=off  SenseRadDot=off  SenseAzimDot=off  SenseDistDot=off  SenseIncDot=off  SenseXDDot=off  SenseYDDot=off  SenseZDDot=off  SenseRadDDot=off  SenseAzimDDot=off  SenseDistDDot=off  SenseIncDDot=off
  World Frame : sm_lib/Frames and Transforms/World Frame
  Frame : PMIOPort  Port=1  Side=Left
  wires:
  Mux/1 -> Kinematic Data/1
  PS-Simulink Converter/1 -> Mux/1
  PS-Simulink Converter1/1 -> Mux/2
  PS-Simulink Converter2/1 -> Mux/3
  PS-Simulink Converter3/1 -> Mux/4
  connections:
  PS-Simulink Converter3/LConn1 -- Transform Sensor/RConn5
  PS-Simulink Converter2/LConn1 -- Transform Sensor/RConn4
  PS-Simulink Converter1/LConn1 -- Transform Sensor/RConn3
  PS-Simulink Converter/LConn1 -- Transform Sensor/RConn2
  Transform Sensor/RConn1 -- Frame/RConn1
  Transform Sensor/LConn1 -- World Frame/RConn1

== system atrias_original/ATRIAS_sim/Mechanical System Layer/Yaw Shaft/Frame Data ==
  Kinematic Data : ToWorkspace  VariableName=boom_yaw_out  SampleTime=sm.output_sample_time
      settings: Save2DSignal=2-D array (concatenate along first dimension)
  Mux : Mux
  PS-Simulink Converter{,1..3} (4 alike) : nesl_utility/PS-Simulink Converter  PhysicalDomain=network_engine_domain  SubClassName=ps_output  LeftPortType=input  RightPortType=output  PseudoPeriodic=off  Frequencies=[]  Unit=1  AffineConversion=off
  Transform Sensor : sm_lib/Frames and Transforms/Transform Sensor  MeasurementFrame=World  SenseAngle=off  SenseAxis=off  SenseAngle1=off  SenseAngle2=off  SenseAngle3=off  SenseQ=on  SenseR=off  SenseOmegaX=off  SenseOmegaY=off  SenseOmegaZ=off  SenseOmega1=off  SenseOmega2=off  SenseOmega3=off  SenseQDot=off  SenseRDot=off  SenseAlphaX=off  SenseAlphaY=off  SenseAlphaZ=off  SenseAlpha1=off  SenseAlpha2=off  SenseAlpha3=off  SenseQDDot=off  SenseRDDot=off  SenseX=on  SenseY=on  SenseZ=on  SenseRad=off  SenseAzim=off  SenseDist=off  SenseInc=off  SenseXDot=off  SenseYDot=off  SenseZDot=off  SenseRadDot=off  SenseAzimDot=off  SenseDistDot=off  SenseIncDot=off  SenseXDDot=off  SenseYDDot=off  SenseZDDot=off  SenseRadDDot=off  SenseAzimDDot=off  SenseDistDDot=off  SenseIncDDot=off
  World Frame : sm_lib/Frames and Transforms/World Frame
  Frame : PMIOPort  Port=1  Side=Left
  wires:
  Mux/1 -> Kinematic Data/1
  PS-Simulink Converter/1 -> Mux/1
  PS-Simulink Converter1/1 -> Mux/2
  PS-Simulink Converter2/1 -> Mux/3
  PS-Simulink Converter3/1 -> Mux/4
  connections:
  PS-Simulink Converter3/LConn1 -- Transform Sensor/RConn5
  PS-Simulink Converter2/LConn1 -- Transform Sensor/RConn4
  PS-Simulink Converter1/LConn1 -- Transform Sensor/RConn3
  PS-Simulink Converter/LConn1 -- Transform Sensor/RConn2
  Transform Sensor/RConn1 -- Frame/RConn1
  Transform Sensor/LConn1 -- World Frame/RConn1

== system atrias_original/control/RC control/Atrias Swing control/Back//Front PD ==
  Desired Position [rad] [back front] : Inport
  Desired Velocity [rad/s] [back front] : Inport  Port=2
  Desired Acceleration [rad/s^2] [back front] : Inport  Port=3
  Measured Position [rad] [back front] : Inport  Port=4
  Measured Velocity [rad/s] [back front] : Inport  Port=5
  Back Tracking : Scope  NumInputPorts=2
  Front Tracking : Scope  NumInputPorts=2
  Kp_SEA_Trajectory : Constant  Value=mc.kp_swing_trajectory
  Kp_SEA_Trajectory1 : Constant  Value=mc.kd_swing_trajectory
  Mux{1..2,12..13} (4 alike) : Mux  Inputs=2
  Product1 : Product
  Product2 : Product
  Reflected Inertia : Gain  Gain=mc.j_motor
  Selector{,1..3} (4 alike) : Selector  InputPortWidth=2  IndexOptions=Index vector (dialog)  Indices=[1]  OutputSizes=1
  Selector{4..7} (4 alike) : Selector  InputPortWidth=2  IndexOptions=Index vector (dialog)  Indices=[2]  OutputSizes=1
  Sum1 : Sum  Inputs=|+-
  Sum2 : Sum
  Sum7 : Sum  Inputs=|+-
  Sum9 : Sum
  Commanded Torque [Nm] [back front] : Outport
  wires:
  Selector7/1 -> Mux1/2
  Selector6/1 -> Mux1/1
  Selector4/1 -> Mux2/1
  Selector5/1 -> Mux2/2
  Selector3/1 -> Mux12/2
  Selector2/1 -> Mux12/1
  Selector1/1 -> Mux13/2
  Selector/1 -> Mux13/1
  Mux2/1 -> Front Tracking/1
  Mux1/1 -> Front Tracking/2
  Desired Position [rad] [back front]/1 -> Sum7/1, Selector1/1, Selector5/1
  Mux13/1 -> Back Tracking/1
  Mux12/1 -> Back Tracking/2
  Product1/1 -> Sum9/1
  Sum7/1 -> Product1/1
  Measured Position [rad] [back front]/1 -> Sum7/2, Selector/1, Selector4/1
  Desired Velocity [rad/s] [back front]/1 -> Sum1/1, Selector2/1, Selector6/1
  Measured Velocity [rad/s] [back front]/1 -> Sum1/2, Selector3/1, Selector7/1
  Sum2/1 -> Commanded Torque [Nm] [back front]/1
  Kp_SEA_Trajectory/1 -> Product1/2
  Kp_SEA_Trajectory1/1 -> Product2/2
  Sum1/1 -> Product2/1
  Product2/1 -> Sum9/2
  Sum9/1 -> Sum2/1
  Desired Acceleration [rad/s^2] [back front]/1 -> Reflected Inertia/1
  Reflected Inertia/1 -> Sum2/2

== system atrias_original/control/RC control/Fz_commanded/Compute Forces1 ==
  XYZ Acceleration : Inport
  Constant5 : Constant  Value=mc.g
  Demux : Demux  Outputs=3
  Gain4 : Gain  Gain=mc.m_total_real
  Mux : Mux  Inputs=3
  Sum8 : Sum  Inputs=|++
  XYZ Force : Outport
  wires:
  Demux/1 -> Mux/1
  Demux/2 -> Mux/2
  Demux/3 -> Sum8/1
  Sum8/1 -> Mux/3
  Mux/1 -> Gain4/1
  Gain4/1 -> XYZ Force/1
  XYZ Acceleration/1 -> Demux/1
  Constant5/1 -> Sum8/2

== system atrias_original/control/RC control/Inverse Dynamics 2D/Leg Force-Torque Distribution ==
  Front Spring Torque [Nm] : Inport
  Back Spring Torque [Nm] : Inport  Port=2
  w [m] : Inport  Port=3
  Compare To Constant : simulink/Logic and Bit Operations/Compare To Constant  relop=<=  const=0.35  OutDataTypeStr=boolean
  Divide : Product  Inputs=*/
  Scope : Scope
  Stop Simulation : Stop  Commented=on
  Sum2 : Sum  Inputs=+|+
  Sum5 : Sum  Inputs=+|-
  Leg Force [N] : Outport
  Leg Torque [Nm] : Outport  Port=2
  wires:
  Divide/1 -> Leg Force [N]/1
  Front Spring Torque [Nm]/1 -> Sum2/1, Sum5/1
  w [m]/1 -> Scope/1, Compare To Constant/1, Divide/2
  Sum5/1 -> Divide/1
  Back Spring Torque [Nm]/1 -> Sum2/2, Sum5/2
  Sum2/1 -> Leg Torque [Nm]/1
  Compare To Constant/1 -> Stop Simulation/1

== system atrias_original/control/RC control/Primary Secondary Leg Swap/Enabled Subsystem ==
  In1 : Inport
  Enable : EnablePort
  Out1 : Outport
  wires:
  In1/1 -> Out1/1

== system atrias_original/control/RC control/State Estimation/Kalman Filtering ==
  "COM from Left Foot [body, yawed, global]" : Inport  SampleTime=sample_time
  "dCOM from Left Foot [body, yawed, global]" : Inport  Port=2  SampleTime=sample_time
  "COM from Right Foot [body, yawed, global]" : Inport  Port=3  SampleTime=sample_time
  "dCOM from Right Foot [body, yawed, global]" : Inport  Port=4  SampleTime=sample_time
  GRFx [N] : Inport  Port=5  SampleTime=sample_time
  GRFz [N] : Inport  Port=6  SampleTime=sample_time
  Right Vertical GRF [N] : Inport  Port=7  SampleTime=sample_time
  Left Vertical GRF [N] : Inport  Port=8  SampleTime=sample_time
  "Initial [x, dx, ddx] [m, m/s, m/s^2]" : Inport  Port=9  PortDimensions=3  SampleTime=sample_time
  "Initial [y, dy, ddy] [m, m/s, m/s^2]" : Inport  Port=10  PortDimensions=3  SampleTime=sample_time
  "Initial [z, dz, ddz] [m m/s m/s^2]" : Inport  Port=11  PortDimensions=3  SampleTime=sample_time
  COM XYZ Acceleration [m/s^2] x3 : Inport  Port=12  SampleTime=sample_time
  Entering Stance [1/0] : Inport  Port=13  PortDimensions=1  SampleTime=sample_time
  Enable : EnablePort  StatesWhenEnabling=reset
  Demux : Demux  Outputs=3
  Difference : simulink/Discrete/Difference  ICPrevInput=0.0  InputProcessing=Inherited  OutMin=[]  OutMax=[]  OutDataType=fixdt(1, 16)  OutScaling=2^-10  DoSatur=off
  Difference1 : simulink/Discrete/Difference  ICPrevInput=0.0  InputProcessing=Inherited  OutMin=[]  OutMax=[]  OutDataType=fixdt(1, 16)  OutScaling=2^-10  DoSatur=off
  Difference2 : simulink/Discrete/Difference  ICPrevInput=0.0  InputProcessing=Inherited  OutMin=[]  OutMax=[]  OutDataType=fixdt(1, 16)  OutScaling=2^-10  DoSatur=off
  GRFs : Scope  NumInputPorts=3
  GRFy : Constant  Value=0
  Logical Operator : Logic  Operator=NOT  AllPortsSameDT=off  OutDataTypeStr=boolean
  Measurement Noise Covariance Matricies : MATLAB Function  TreatAsAtomicUnit=on
  Mux{,1,3,5} (4 alike) : Mux  Inputs=3
  Mux2 : Mux  Inputs=2
  P0_kalman_transverse : Constant  Value=mc.P0_kalman_transverse
  P0_kalman_transverse1 : Constant  Value=mc.P0_kalman_transverse
  P0_kalman_transverse2 : Constant  Value=mc.P0_kalman_no_position
  P0_kalman_vertical : Constant  Value=mc.P0_kalman_vertical
  Product : Product
  Product1 : Product
  Product2 : Product
  Rt : Scope  NumInputPorts=2
  Selector : Selector  InputPortWidth=3  IndexOptions=Index vector (dialog)  Indices=[1]  OutputSizes=1
  Selector4 : Selector  InputPortWidth=3  IndexOptions=Index vector (dialog)  Indices=[2 3]  OutputSizes=1
  Terminator : Terminator
  X Kalman Output : Scope  NumInputPorts=3
  X State Kalman Filter : ctrlSharedLib/Kalman Filter  TimeDomain=Discrete-Time  UseCurrentEstimator=on  ModelSource=Individual A, B, C, D matrices  ModelSourceVariable=A_kf  A=mc.A_kalman_transverse  B=mc.B_kalman_transverse  C=mc.C_kalman_transverse  D=0  NumberOfStates=2  NumberOfInputs=1  NumberOfOutputs=2  InitialEstimateSource=Input port  X0=initial_dx_estimate  P0=P0_kalman_transverse  UseK=off  UseGH=on  NumberOfProcessNoiseInputs=1  G=mc.G_kalman_transverse  TimeInvariantG=on  H=0  TimeInvariantH=on  Q=mc.Q_kalman_GRFx_difference*sample_time  TimeInvariantQ=on  R=1  TimeInvariantR=off  N=0  TimeInvariantN=on  AddInputPort=on  AddEnablePort=off  ExternalReset=Rising  OutputEstimatedY=off  OutputP=on  Ts=sample_time
  Y State Kalman Filter : ctrlSharedLib/Kalman Filter  TimeDomain=Discrete-Time  UseCurrentEstimator=on  ModelSource=Individual A, B, C, D matrices  ModelSourceVariable=A_kf  A=mc.A_kalman_transverse  B=mc.B_kalman_transverse  C=mc.C_kalman_transverse  D=0  NumberOfStates=2  NumberOfInputs=1  NumberOfOutputs=2  InitialEstimateSource=Input port  X0=initial_dy_estimate  P0=P0_kalman_transverse  UseK=off  UseGH=on  NumberOfProcessNoiseInputs=1  G=mc.G_kalman_transverse  TimeInvariantG=on  H=0  TimeInvariantH=on  Q=mc.Q_kalman_GRFy_difference*sample_time  TimeInvariantQ=on  R=1  TimeInvariantR=off  N=0  TimeInvariantN=on  AddInputPort=on  AddEnablePort=off  ExternalReset=Rising  OutputEstimatedY=off  OutputP=on  Ts=sample_time
  Z State Kalman Filter : ctrlSharedLib/Kalman Filter  TimeDomain=Discrete-Time  UseCurrentEstimator=on  ModelSource=Individual A, B, C, D matrices  ModelSourceVariable=A_kf  A=mc.A_kalman_vertical  B=mc.B_kalman_vertical  C=mc.C_kalman_vertical  D=0  NumberOfStates=2  NumberOfInputs=1  NumberOfOutputs=2  InitialEstimateSource=Input port  X0=[initial_z_estimate; initial_dz_estimate]  P0=P0_kalman_vertical  UseK=off  UseGH=on  NumberOfProcessNoiseInputs=1  G=mc.G_kalman_vertical  TimeInvariantG=on  H=0  TimeInvariantH=on  Q=mc.Q_kalman_GRFz_difference*sample_time  TimeInvariantQ=on  R=1  TimeInvariantR=off  N=0  TimeInvariantN=on  AddInputPort=on  AddEnablePort=off  OutputEstimatedY=off  OutputP=on  Ts=sample_time
  "dX, ddX Kalman Filter" : ctrlSharedLib/Kalman Filter  TimeDomain=Discrete-Time  UseCurrentEstimator=on  ModelSource=Individual A, B, C, D matrices  ModelSourceVariable=A_kf  A=mc.A_kalman_no_position  B=mc.B_kalman_no_position  C=mc.C_kalman_no_position  D=0  NumberOfStates=2  NumberOfInputs=1  NumberOfOutputs=2  InitialEstimateSource=Input port  X0=initial_dx_estimate  P0=P0_kalman_transverse  UseK=off  UseGH=on  NumberOfProcessNoiseInputs=1  G=mc.G_kalman_no_position  TimeInvariantG=on  H=0  TimeInvariantH=on  Q=mc.Q_kalman_GRFx_difference*sample_time  TimeInvariantQ=on  R=1  TimeInvariantR=off  N=0  TimeInvariantN=on  AddInputPort=on  AddEnablePort=off  OutputEstimatedY=off  OutputP=on  Ts=sample_time
  eigen values : MATLAB Function  TreatAsAtomicUnit=on
  eigen values1 : MATLAB Function  TreatAsAtomicUnit=on
  eigen values2 : MATLAB Function  TreatAsAtomicUnit=on
  left dx yawed : Selector  InputPortWidth=9  IndexOptions=Index vector (dialog)  Indices=[4]  OutputSizes=1
  left x yawed : Selector  InputPortWidth=9  IndexOptions=Index vector (dialog)  Indices=[4]  OutputSizes=1
  left y yawed : Selector  InputPortWidth=9  IndexOptions=Index vector (dialog)  Indices=[5]  OutputSizes=1
  left z yawed : Selector  InputPortWidth=9  IndexOptions=Index vector (dialog)  Indices=[6]  OutputSizes=1
  right dx yawed : Selector  InputPortWidth=9  IndexOptions=Index vector (dialog)  Indices=[4]  OutputSizes=1
  right x yawed : Selector  InputPortWidth=9  IndexOptions=Index vector (dialog)  Indices=[4]  OutputSizes=1
  right y yawed : Selector  InputPortWidth=9  IndexOptions=Index vector (dialog)  Indices=[5]  OutputSizes=1
  right z yawed : Selector  InputPortWidth=9  IndexOptions=Index vector (dialog)  Indices=[6]  OutputSizes=1
  x acceleration : Selector  InputPortWidth=3  IndexOptions=Index vector (dialog)  Indices=[1]  OutputSizes=1
  y acceleration : Selector  InputPortWidth=3  IndexOptions=Index vector (dialog)  Indices=[2]  OutputSizes=1
  z acceleration : Selector  InputPortWidth=3  IndexOptions=Index vector (dialog)  Indices=[3]  OutputSizes=1
  "[x, dx, ddx] [m/s, m/s^2]" : Outport
  "[y, dy, ddy] [m/s, m/s^2]" : Outport  Port=2
  "[z, dz, ddz] [m, m/s, m/s^2]" : Outport  Port=3
  "[x, dx, ddx] uncertainty" : Outport  Port=4
  "[y, dy, ddy] uncertainty" : Outport  Port=5
  "[z, dz, ddz] uncertainty" : Outport  Port=6
  wires:
  Measurement Noise Covariance Matricies/2(R_transverse) -> X State Kalman Filter/6, Y State Kalman Filter/6
  "dX, ddX Kalman Filter"/2 -> Terminator/1
  Mux2/1 -> "[x, dx, ddx] [m/s, m/s^2]"/1
  "dX, ddX Kalman Filter"/1 -> Mux2/2
  Selector/1 -> Mux2/1
  X State Kalman Filter/1 -> Selector/1
  Product2/1 -> X State Kalman Filter/1, "dX, ddX Kalman Filter"/1
  P0_kalman_transverse/1 -> X State Kalman Filter/4
  GRFz [N]/1 -> Difference/1
  Product/1 -> Z State Kalman Filter/1
  Product1/1 -> Y State Kalman Filter/1
  Difference2/1 -> Product2/2
  Difference1/1 -> Product1/2
  Entering Stance [1/0]/1 -> X State Kalman Filter/5, Y State Kalman Filter/5, Logical Operator/1
  Difference/1 -> Product/2
  Logical Operator/1 -> Product2/1, Product1/1, Product/1
  eigen values/1(E) -> "[z, dz, ddz] uncertainty"/1
  Z State Kalman Filter/2 -> eigen values/1(Z)
  Y State Kalman Filter/2 -> eigen values1/1(Z)
  X State Kalman Filter/2 -> eigen values2/1(Z)
  "Initial [z, dz, ddz] [m m/s m/s^2]"/1 -> Z State Kalman Filter/3
  P0_kalman_vertical/1 -> Z State Kalman Filter/4
  "Initial [y, dy, ddy] [m, m/s, m/s^2]"/1 -> Y State Kalman Filter/3
  P0_kalman_transverse1/1 -> Y State Kalman Filter/4
  "Initial [x, dx, ddx] [m, m/s, m/s^2]"/1 -> X State Kalman Filter/3, Selector4/1
  right z yawed/1 -> Mux3/2
  left z yawed/1 -> Mux3/1
  right y yawed/1 -> Mux1/2
  left y yawed/1 -> Mux1/1
  right x yawed/1 -> Mux/2
  "COM from Right Foot [body, yawed, global]"/1 -> right x yawed/1, right y yawed/1, right z yawed/1
  left x yawed/1 -> Mux/1
  "COM from Left Foot [body, yawed, global]"/1 -> left x yawed/1, left y yawed/1, left z yawed/1
  Left Vertical GRF [N]/1 -> GRFs/1, Measurement Noise Covariance Matricies/1(vertical_GRF_L)
  Right Vertical GRF [N]/1 -> GRFs/2, Measurement Noise Covariance Matricies/2(vertical_GRF_R)
  Mux/1 -> X State Kalman Filter/2  "yawed [left x, right x, ddx]"
  Mux1/1 -> Y State Kalman Filter/2  "yawed [left y, right y, ddy]"
  Measurement Noise Covariance Matricies/3(R_vertical) -> Z State Kalman Filter/5
  GRFx [N]/1 -> GRFs/3, Difference2/1
  Mux3/1 -> Z State Kalman Filter/2  "yawed [left z, right z, ddz]"
  GRFy/1 -> Difference1/1
  Z State Kalman Filter/1 -> "[z, dz, ddz] [m, m/s, m/s^2]"/1
  COM XYZ Acceleration [m/s^2] x3/1 -> x acceleration/1, y acceleration/1, z acceleration/1
  x acceleration/1 -> Mux5/3, Mux/3
  y acceleration/1 -> Mux1/3
  Y State Kalman Filter/1 -> "[y, dy, ddy] [m/s, m/s^2]"/1
  eigen values2/1(E) -> Demux/1, "[x, dx, ddx] uncertainty"/1
  eigen values1/1(E) -> "[y, dy, ddy] uncertainty"/1
  left dx yawed/1 -> Mux5/1
  right dx yawed/1 -> Mux5/2
  Mux5/1 -> "dX, ddX Kalman Filter"/2
  Selector4/1 -> "dX, ddX Kalman Filter"/3
  P0_kalman_transverse2/1 -> "dX, ddX Kalman Filter"/4
  Measurement Noise Covariance Matricies/1(R_no_position) -> "dX, ddX Kalman Filter"/5
  "dCOM from Left Foot [body, yawed, global]"/1 -> left dx yawed/1
  "dCOM from Right Foot [body, yawed, global]"/1 -> right dx yawed/1
  z acceleration/1 -> Mux3/3
  Demux/1 -> X Kalman Output/1
  Demux/2 -> X Kalman Output/2
  Demux/3 -> X Kalman Output/3
  Measurement Noise Covariance Matricies/4(R_t_L) -> Rt/1
  Measurement Noise Covariance Matricies/5(R_t_R) -> Rt/2

== system atrias_original/control/RC control/Swing/Enabled Subsystem ==
  In1 : Inport
  Enable : EnablePort
  Out1 : Outport
  wires:
  In1/1 -> Out1/1

== system atrias_original/control/RC control/Swing/Hold Value1 ==
  In1 : Inport
  Enable : EnablePort
  Out1 : Outport  InitialOutput=0.25
  wires:
  In1/1 -> Out1/1

== system atrias_original/control/RC control/lateral_PID_control/Lateral Hip PID1 ==
  position_error : Inport
  velocity_error : Inport  Port=2
  Proportional Gain : Gain  Description=xPCTag(1)=kp_lateral;  Gain=mc.kp_lateral
  Proportional Gain1 : Gain  Description=xPCTag(1)=kd_lateral;  Gain=mc.kd_lateral
  Sum : Sum  Inputs=++|
  out : Outport
  wires:
  velocity_error/1 -> Proportional Gain1/1
  Proportional Gain/1 -> Sum/2
  position_error/1 -> Proportional Gain/1
  Sum/1 -> out/1
  Proportional Gain1/1 -> Sum/1

== system atrias_original/control/RC control/lateral_PID_control/Swing Leg Lateral ==
  position_error : Inport
  velocity_error : Inport  Port=2
  Proportional Gain : Gain  Description=xPCTag(1)=kp_lateral;  Gain=mc.kp_lateral
  Proportional Gain1 : Gain  Description=xPCTag(1)=kd_lateral;  Gain=mc.kd_lateral
  Sum : Sum  Inputs=++|
  out : Outport
  wires:
  Proportional Gain1/1 -> Sum/1
  Sum/1 -> out/1
  position_error/1 -> Proportional Gain/1
  Proportional Gain/1 -> Sum/2
  velocity_error/1 -> Proportional Gain1/1

== system atrias_original/control/RC control/lateral_PID_control/spherical_correction_angle ==
  q_boom_roll : Inport
  Sum1 : Sum  Inputs=|+-
  boom_mount_angle : Constant  Value=mc.boom_mount_angle
  lateral_correction [rad] : Outport
  wires:
  boom_mount_angle/1 -> Sum1/2
  q_boom_roll/1 -> Sum1/1
  Sum1/1 -> lateral_correction [rad]/1

== system atrias_original/control/Robot-to-NMM Interface/Force Estimation/Horizontal GRF ==
  Axial Force [N] : Inport
  Orthogonal Force [N] : Inport  Port=2
  Torso Pitch [rad] : Inport  Port=3
  Leg Angle [rad] : Inport  Port=4
  Gain : Gain  Gain=-1
  Gain1 : Gain  Gain=-1
  Product : Product
  Product1 : Product
  Sum : Sum  Inputs=++|
  Sum1 : Sum  Inputs=+|+
  Trigonometric Function : Trigonometry
  Trigonometric Function1 : Trigonometry  Operator=cos
  Horizontal Force [N] : Outport
  wires:
  Product1/1 -> Gain/1
  Sum1/1 -> Horizontal Force [N]/1
  Trigonometric Function1/1 -> Product1/2
  Orthogonal Force [N]/1 -> Product1/1
  Axial Force [N]/1 -> Product/1
  Leg Angle [rad]/1 -> Sum/2
  Torso Pitch [rad]/1 -> Sum/1
  Trigonometric Function/1 -> Product/2
  Sum/1 -> Trigonometric Function/1, Trigonometric Function1/1
  Product/1 -> Gain1/1
  Gain/1 -> Sum1/2
  Gain1/1 -> Sum1/1

== system atrias_original/control/Robot-to-NMM Interface/Force Estimation/Leg Force Measurements ==
  q : Inport
  Leg Width Right/Left [m m] : Inport  Port=2
  Leg Length Right/Left [m m] : Inport  Port=3
  Demux : Demux  Outputs=2
  Demux1 : Demux  Outputs=2
  Demux2 : Demux
  Divide{1..4} (4 alike) : Product  Inputs=*/
  Gain : Gain  Gain=3500
  Mux : Mux
  Nonlinear Spring Force : MATLAB Function  Commented=on  TreatAsAtomicUnit=on
  Sum{1..3,6} (4 alike) : Sum  Inputs=-+|
  Sum4 : Sum  Inputs=-|+
  Sum5 : Sum  Inputs=-|+
  Sum7 : Sum  Inputs=+|+
  Sum8 : Sum  Inputs=+|+
  backGearL : Selector  InputPortWidth=13  IndexOptions=Index vector (dialog)  Indices=[6]  OutputSizes=1
  backGearR : Selector  InputPortWidth=13  IndexOptions=Index vector (dialog)  Indices=[2]  OutputSizes=1
  backJointL : Selector  InputPortWidth=13  IndexOptions=Index vector (dialog)  Indices=[5]  OutputSizes=1
  backJointR : Selector  InputPortWidth=13  IndexOptions=Index vector (dialog)  Indices=[1]  OutputSizes=1
  frontGearL : Selector  InputPortWidth=13  IndexOptions=Index vector (dialog)  Indices=[8]  OutputSizes=1
  frontGearR : Selector  InputPortWidth=13  IndexOptions=Index vector (dialog)  Indices=[4]  OutputSizes=1
  frontJointL : Selector  InputPortWidth=13  IndexOptions=Index vector (dialog)  Indices=[7]  OutputSizes=1
  frontJointR : Selector  InputPortWidth=13  IndexOptions=Index vector (dialog)  Indices=[3]  OutputSizes=1
  Right Leg Torque [Nm] : Outport
  Left Leg Torque [Nm] : Outport  Port=2
  Right Leg Axial Force [N] : Outport  Port=3
  Left Leg Axial Force [N] : Outport  Port=4
  Right Leg Orthogonal Force [N] : Outport  Port=5
  Left Leg Orthogonal Force [N] : Outport  Port=6
  wires:
  Sum3/1 -> Mux/4
  Sum2/1 -> Mux/3
  backJointL/1 -> Sum2/1
  frontGearL/1 -> Sum3/2
  frontJointL/1 -> Sum3/1
  backGearL/1 -> Sum2/2
  Sum6/1 -> Mux/1
  Sum1/1 -> Mux/2
  backJointR/1 -> Sum6/1
  frontGearR/1 -> Sum1/2
  frontJointR/1 -> Sum1/1
  backGearR/1 -> Sum6/2
  q/1 -> backGearR/1, backJointL/1, frontJointL/1, frontGearL/1, backGearL/1, frontGearR/1, frontJointR/1, backJointR/1
  Demux2/1 -> Sum4/1, Sum7/1
  Demux2/2 -> Sum7/2, Sum4/2
  Demux2/4 -> Sum5/2, Sum8/2
  Sum4/1 -> Divide1/1
  Sum5/1 -> Divide2/1
  Leg Width Right/Left [m m]/1 -> Demux/1
  Demux/1 -> Divide1/2
  Demux/2 -> Divide2/2
  Divide1/1 -> Right Leg Axial Force [N]/1
  Divide2/1 -> Left Leg Axial Force [N]/1
  Demux2/3 -> Sum8/1, Sum5/1
  Sum7/1 -> Divide3/1, Right Leg Torque [Nm]/1
  Sum8/1 -> Divide4/1, Left Leg Torque [Nm]/1
  Demux1/1 -> Divide3/2
  Demux1/2 -> Divide4/2
  Leg Length Right/Left [m m]/1 -> Demux1/1
  Divide3/1 -> Right Leg Orthogonal Force [N]/1
  Divide4/1 -> Left Leg Orthogonal Force [N]/1
  Mux/1 -> Gain/1
  Gain/1 -> Demux2/1
